simulink model "BANSHEE"  (Simulink 8.7)
settings: Solver=ode1  StartTime=0.0  StopTime=inf  FixedStep=Ts  MaxStep=1e-3  RelTol=1e-3
PostLoadFcn:
  | BANSHEE_init;
InitFcn:
  | BANSHEE_init;
values from neighbouring files (symbols this model uses):
  Ts = 100E-6    (= 0.0001)    [BANSHEE_init.m]
undefined symbols (not defined in the file or in its folder): Acid, Banshee_HWCtrl_IOs, Banshee_SEL751_Woodward_lib, DMS_slave_lib, DMSCommands, F1, F2, F3, fdesignblkfcn, Feeder1_lib, Feeder2_lib, Feeder3_lib, gcbh, generic_ethernet_cb, Lead, Left, relay_housing_lib, SM_UtilityService, SS_F1_RELAY_HOUSING, SS_F2_RELAY_HOUSING, SS_F3_RELAY_HOUSING, SS_Feeder1, SS_Feeder2, SS_Feeder3, SUBSTATION, TestSeq_slave_lib, TestSequenceCommands, type, utility_service_lib, V
libraries: powerlib x108, cables_lib x61, breaker_lib x53, rtio_generic_modbus x50, relay_modbus_lib x45, rtio_opalrt_op5142ex1 x37, transformer_lib x29, rteventslib x28, Load_lib x25, simulink x24, rtlab x20, ssn_lib x19
(part 6 of 9)

== system BANSHEE/SM_UtilityService/Banshee_HWCtrl_IOs/SEL-2440 FAST-LOAD-SHEDDING AND CB STATUS ==
  note: Breaker status
  note: CB202
      | CB203
      | CB301
      | CB302
      | CB303
      | CB304
      | spare
      | spare
  note: 751-1
      | 751-2
      | 751-3
      | CB101
      | CB102
      | CB103
      | CB108
      | CB201
  note: CB204
      | CB307
      | CB218
      | CB309
      | F1-GCB
      | CB205
      | CB211
      | F3-GCB
  note: CB104
      | CB107
      | CB206
      | CB208
      | CB212
      | CB308
      | CB114
      | CB219
  note: Copyright (c) 2016 Massachusetts Institute of Technology
      | Permission is hereby granted, free of charge, to any person obtaining a copy of this software and associated documentation files (the "Software"), to deal
      | in the Software without restriction, including without limitation the rights to use, copy, modify, merge, publish, distribute, sublicense, and/or sell copies of the
      | Software, and to permit persons to whom the Software is furnished to do so, subject to the following conditions:
      |
      | THE SOFTWARE IS PROVIDED "AS IS", WITHOUT WARRANTY OF ANY KIND, EXPRESS OR IMPLIED, INCLUDING BUT NOT LIMITED TO THE
      | WARRANTIES OF MERCHANTABILITY, FITNESS FOR A PARTICULAR PURPOSE AND NONINFRINGEMENT. IN NO EVENT SHALL THE AUTHORS
      | OR COPYRIGHT HOLDERS BE LIABLE FOR ANY CLAIM, DAMAGES OR OTHER LIABILITY, WHETHER IN AN ACTION OF CONTRACT, TORT OR
      | OTHERWISE, ARISING FROM, OUT OF OR IN CONNECTION WITH THE SOFTWARE OR THE USE OR OTHER DEALINGS IN THE SOFTWARE
  note: 16 bits to control (P, I load) breakers from Schwietzer
  CMBNE_SGNLS : Inport
  Bus Creator : BusCreator  Inputs=16
  Bus Selector : BusSelector  OutputSignals=F1_MS_IN.CB_DATA.F1_CB_4.Status,F1_MS_IN.CB_DATA.F1_CB_7.Status,F2_MS_IN.CB_DATA.F2_CB_6.Status,F2_MS_IN.CB_DATA.F2_CB_8.Status,F2_MS_IN.CB_DATA.F2_CB_12.Status,F3_MS_IN.CB_DATA.F3_CB_8.Status,F1_MS_IN.CB_DATA.F1_CB_14.Status,F2_MS_IN.CB_DATA.F2_CB_19.Status  OutputAsBus=on
  Bus Selector1 : BusSelector  OutputSignals=BESS_PV.EPC.BESS.BESS_MX1.cb_ms.Status,BESS_PV.EPC.PV.PV_MX1.cb_ms.Status
  Bus Selector6 : BusSelector  OutputSignals=F2_MS_IN.CB_DATA.F2_CB_4.Status,F3_MS_IN.CB_DATA.F3_CB_7.Status,F2_MS_IN.CB_DATA.F2_CB_18.Status,F3_MS_IN.CB_DATA.F3_CB_9.Status,F1_MS_IN.DIESEL_DATA.DIESEL_GCB.cb_ms.Status,F2_MS_IN.CB_DATA.F2_CB_5.Status,F2_MS_IN.CB_DATA.F2_CB_11.Status,F3_MS_IN.NG_CHP_DATA.NG_CHP_GCB.cb_ms.Status
  Bus Selector7 : BusSelector  OutputSignals=F1_MS_IN.CB_DATA.F1_PCC.Status,F2_MS_IN.CB_DATA.F2_PCC.Status,F3_MS_IN.CB_DATA.F3_PCC.Status,F1_MS_IN.CB_DATA.F1_CB_1.Status,F1_MS_IN.CB_DATA.F1_CB_2.Status,F1_MS_IN.CB_DATA.F1_CB_3.Status,F1_MS_IN.CB_DATA.F1_CB_8.Status,F2_MS_IN.CB_DATA.F2_CB_1.Status  OutputAsBus=on
  Bus Selector8 : BusSelector  OutputSignals=F2_MS_IN.CB_DATA.F2_CB_2.Status,F2_MS_IN.CB_DATA.F2_CB_3.Status,F3_MS_IN.CB_DATA.F3_CB_1.Status,F3_MS_IN.CB_DATA.F3_CB_2.Status,F3_MS_IN.CB_DATA.F3_CB_3.Status,F3_MS_IN.CB_DATA.F3_CB_4.Status
  Data Type Conversion : DataTypeConversion
  Data Type Conversion1 : DataTypeConversion
  Demux : Demux  Outputs=8
  Demux1 : Demux  Outputs=8
  Logical Operator : Logic  AllPortsSameDT=off  OutDataTypeStr=boolean
  Logical Operator1 : Logic  AllPortsSameDT=off  OutDataTypeStr=boolean
  Mux1 : Mux  Inputs=8
  Mux3 : Mux  Inputs=8
  OP5142EX1 DigitalIn : rtio_opalrt_op5142ex1/OP5142EX1 DigitalIn  CtrlName='OP5142EX1 Ctrl'  portNb=3  FcnNos=Slot 4 Module A Subsection 1  size=1  maxcount=8  count=8  sampleTime=0  numchan=8
      settings: AttributesFormatString=%<CtrlName>
  OP5142EX1 DigitalIn1 : rtio_opalrt_op5142ex1/OP5142EX1 DigitalIn  CtrlName='OP5142EX1 Ctrl'  portNb=4  FcnNos=Slot 4 Module A Subsection 2  size=1  maxcount=8  count=8  sampleTime=0  numchan=8
      settings: AttributesFormatString=%<CtrlName>
  OP5142EX1 DigitalOut : rtio_opalrt_op5142ex1/OP5142EX1 DigitalOut  CtrlName='OP5142EX1 Ctrl'  portNb=9  FcnNos=Slot 3 Module B Subsection 1  size=1  maxcount=8  count=8  numchan=8
      settings: AttributesFormatString=%<CtrlName>
  OP5142EX1 DigitalOut1 : rtio_opalrt_op5142ex1/OP5142EX1 DigitalOut  CtrlName='OP5142EX1 Ctrl'  portNb=10  FcnNos=Slot 3 Module B Subsection 2  size=1  maxcount=8  count=8  numchan=8
      settings: AttributesFormatString=%<CtrlName>
  OP5142EX1 DigitalOut2 : rtio_opalrt_op5142ex1/OP5142EX1 DigitalOut  CtrlName='OP5142EX1 Ctrl'  portNb=11  FcnNos=Slot 3 Module B Subsection 3  size=1  maxcount=8  count=8  numchan=8
      settings: AttributesFormatString=%<CtrlName>
  OP5142EX1 DigitalOut3 : rtio_opalrt_op5142ex1/OP5142EX1 DigitalOut  CtrlName='OP5142EX1 Ctrl'  portNb=12  FcnNos=Slot 3 Module B Subsection 4  size=1  maxcount=8  count=8  numchan=8
      settings: AttributesFormatString=%<CtrlName>
  Spares : Constant  Value=0
  Terminator1 : Terminator
  Terminator7 : Terminator
  SEL2440_FLS : Outport
  wires:
  [CMBNE_SGNLS] -> Bus Selector/1
  Bus Selector/1 -> OP5142EX1 DigitalOut/1
  Bus Selector8/1 -> Mux3/1  "<Status>"
  Bus Selector8/3 -> Mux3/3  "<Status>"
  Bus Selector8/2 -> Mux3/2  "<Status>"
  Bus Selector8/5 -> Mux3/5  "<Status>"
  Spares/1 -> Mux3/7, Mux3/8
  Bus Selector8/4 -> Mux3/4  "<Status>"
  Bus Selector7/1 -> OP5142EX1 DigitalOut2/1
  Bus Selector8/6 -> Mux3/6  "<Status>"
  Mux3/1 -> OP5142EX1 DigitalOut3/1
  OP5142EX1 DigitalIn/2 -> Terminator7/1
  OP5142EX1 DigitalIn1/2 -> Terminator1/1
  OP5142EX1 DigitalIn/1 -> Demux/1
  OP5142EX1 DigitalIn1/1 -> Demux1/1
  Demux/1 -> Bus Creator/1  "CB104"
  Demux/2 -> Bus Creator/2  "CB107"
  Demux/3 -> Bus Creator/3  "CB206"
  Demux/4 -> Bus Creator/4  "CB208"
  Demux/5 -> Bus Creator/5  "CB212"
  Demux/6 -> Bus Creator/6  "CB308"
  Demux/7 -> Bus Creator/7  "CB114"
  Demux/8 -> Bus Creator/8  "CB219"
  Demux1/7 -> Bus Creator/15
  Demux1/8 -> Bus Creator/16
  Demux1/6 -> Bus Creator/14
  Demux1/5 -> Bus Creator/13
  Demux1/4 -> Bus Creator/12  "CB309"
  Demux1/3 -> Bus Creator/11  "CB218"
  Demux1/2 -> Bus Creator/10  "CB307"
  Demux1/1 -> Bus Creator/9  "CB204"
  Bus Creator/1 -> SEL2440_FLS/1  "SEL2440_FLS"
  CMBNE_SGNLS/1 -> [CMBNE_SGNLS]
  [CMBNE_SGNLS] -> Bus Selector6/1
  [CMBNE_SGNLS] -> Bus Selector7/1
  [CMBNE_SGNLS] -> Bus Selector8/1
  [CMBNE_SGNLS] -> Bus Selector1/1
  Bus Selector1/1 -> [BESS_MX1_Status]  "<Status>"
  Bus Selector1/2 -> [PV_MX1_Status]  "<Status>"
  Bus Selector6/7 -> Logical Operator1/2  "<Status>"
  [PV_MX1_Status] -> Logical Operator1/1
  Bus Selector6/6 -> Logical Operator/2  "<Status>"
  [BESS_MX1_Status] -> Logical Operator/1
  Bus Selector6/5 -> Mux1/5  "<Status>"
  Bus Selector6/4 -> Mux1/4  "<Status>"
  Bus Selector6/3 -> Mux1/3  "<Status>"
  Bus Selector6/2 -> Mux1/2  "<Status>"
  Bus Selector6/1 -> Mux1/1  "<Status>"
  Logical Operator/1 -> Data Type Conversion/1
  Logical Operator1/1 -> Data Type Conversion1/1
  Bus Selector6/8 -> Mux1/8  "<Status>"
  Mux1/1 -> OP5142EX1 DigitalOut1/1
  Data Type Conversion/1 -> Mux1/6
  Data Type Conversion1/1 -> Mux1/7

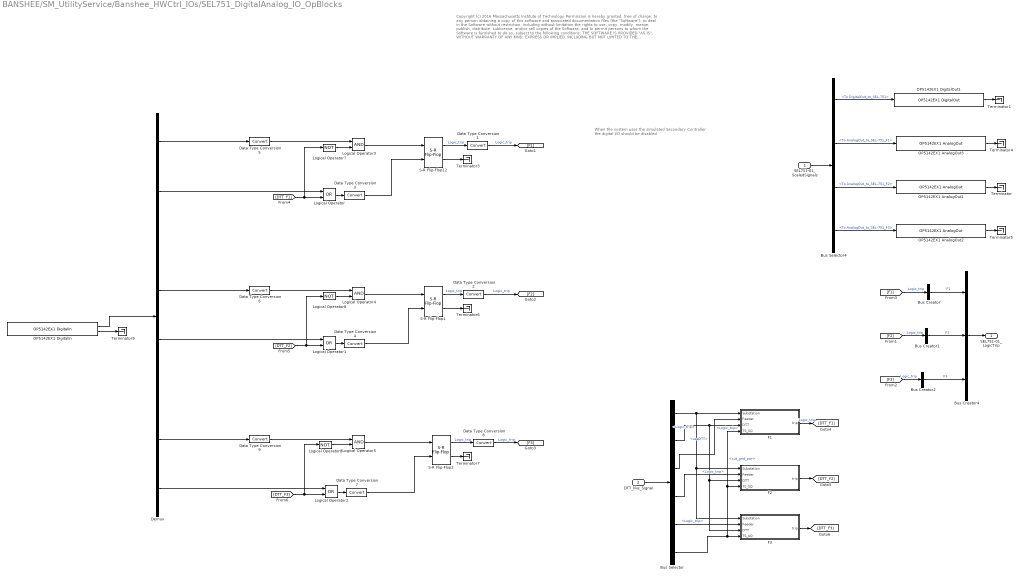
== system BANSHEE/SM_UtilityService/Banshee_HWCtrl_IOs/SEL751_DigitalAnalog_IO_OpBlocks ==
  note: When the system uses the simulated
      | Secondary Controller the digital I/O
      | should be disabled.
  note: Copyright (c) 2016 Massachusetts Institute of Technology
      | Permission is hereby granted, free of charge, to any person obtaining a copy of this software and associated documentation files (the "Software"), to deal
      | in the Software without restriction, including without limitation the rights to use, copy, modify, merge, publish, distribute, sublicense, and/or sell copies of the
      | Software, and to permit persons to whom the Software is furnished to do so, subject to the following conditions:
      |
      | THE SOFTWARE IS PROVIDED "AS IS", WITHOUT WARRANTY OF ANY KIND, EXPRESS OR IMPLIED, INCLUDING BUT NOT LIMITED TO THE
      | WARRANTIES OF MERCHANTABILITY, FITNESS FOR A PARTICULAR PURPOSE AND NONINFRINGEMENT. IN NO EVENT SHALL THE AUTHORS
      | OR COPYRIGHT HOLDERS BE LIABLE FOR ANY CLAIM, DAMAGES OR OTHER LIABILITY, WHETHER IN AN ACTION OF CONTRACT, TORT OR
      | OTHERWISE, ARISING FROM, OUT OF OR IN CONNECTION WITH THE SOFTWARE OR THE USE OR OTHER DEALINGS IN THE SOFTWARE
  SEL751-01_ScaledSignals : Inport
  DTT_like_Signal : Inport  Port=2
  Bus Creator : BusCreator  Inputs=1
  Bus Creator1 : BusCreator  Inputs=1
  Bus Creator2 : BusCreator  Inputs=1
  Bus Creator4 : BusCreator  Inputs=3
  Bus Selector : BusSelector  OutputSignals=SC_Signal.GridStatusCtrl.Substation.Logic_trip,SC_Signal.GridStatusCtrl.useDTT,SC_Signal.GridStatusCtrl.Grid_F1.Logic_trip,SC_Signal.GridStatusCtrl.Grid_F2.Logic_trip,SC_Signal.GridStatusCtrl.Grid_F3.Logic_trip,cut_grid_pwr
  Bus Selector4 : BusSelector  OutputSignals=To DigitalOut_to_SEL-751,To AnalogOut_to_SEL-751_F1,To AnalogOut_to_SEL-751_F2,To AnalogOut_to_SEL-751_F3
  Data Type Conversion{1..9} (9 alike) : DataTypeConversion
  Demux : Demux  Outputs=8
  F1 : Subsystem
  F2 : Subsystem
  F3 : Subsystem
  Logical Operator : Logic  Operator=OR  AllPortsSameDT=off  OutDataTypeStr=boolean
  Logical Operator1 : Logic  Operator=OR  AllPortsSameDT=off  OutDataTypeStr=boolean
  Logical Operator2 : Logic  Operator=OR  AllPortsSameDT=off  OutDataTypeStr=boolean
  Logical Operator3 : Logic  AllPortsSameDT=off  OutDataTypeStr=boolean
  Logical Operator4 : Logic  AllPortsSameDT=off  OutDataTypeStr=boolean
  Logical Operator5 : Logic  AllPortsSameDT=off  OutDataTypeStr=boolean
  Logical Operator6 : Logic  Operator=NOT  AllPortsSameDT=off  OutDataTypeStr=boolean
  Logical Operator7 : Logic  Operator=NOT  AllPortsSameDT=off  OutDataTypeStr=boolean
  Logical Operator8 : Logic  Operator=NOT  AllPortsSameDT=off  OutDataTypeStr=boolean
  OP5142EX1 AnalogOut1 : rtio_opalrt_op5142ex1/OP5142EX1 AnalogOut  CtrlName='OP5142EX1 Ctrl'  portNb=2  FcnNos=Slot 1 Module A Subsection 2  size=16  maxcount=8  count=8  numchan=8  israngeinput=off  voltagerange=[-16 ... 16]  slot=0  side=0  mismatch=0  slotside=Slot_1_Module_A
      settings: AttributesFormatString=%<CtrlName>
  OP5142EX1 AnalogOut2 : rtio_opalrt_op5142ex1/OP5142EX1 AnalogOut  CtrlName='OP5142EX1 Ctrl'  portNb=3  FcnNos=Slot 2 Module A Subsection 1  size=16  maxcount=8  count=8  numchan=8  israngeinput=off  voltagerange=[-16 ... 16]  slot=1  side=0  mismatch=0  slotside=Slot_2_Module_A
      settings: AttributesFormatString=%<CtrlName>
  OP5142EX1 AnalogOut3 : rtio_opalrt_op5142ex1/OP5142EX1 AnalogOut  CtrlName='OP5142EX1 Ctrl'  portNb=1  FcnNos=Slot 1 Module A Subsection 1  size=16  maxcount=8  count=8  numchan=8  israngeinput=off  voltagerange=[-16 ... 16]  slot=0  side=0  mismatch=0  slotside=Slot_1_Module_A
      settings: AttributesFormatString=%<CtrlName>
  OP5142EX1 DigitalIn : rtio_opalrt_op5142ex1/OP5142EX1 DigitalIn  CtrlName='OP5142EX1 Ctrl'  portNb=5  FcnNos=Slot 4 Module A Subsection 3  size=1  maxcount=8  count=8  sampleTime=0  numchan=8
      settings: AttributesFormatString=%<CtrlName>
  OP5142EX1 DigitalOut1 : rtio_opalrt_op5142ex1/OP5142EX1 DigitalOut  CtrlName='OP5142EX1 Ctrl'  portNb=13  FcnNos=Slot 4 Module B Subsection 1  size=1  maxcount=8  count=8  numchan=8
      settings: AttributesFormatString=%<CtrlName>
  S-R Flip-Flop1 : simulink_extras/Flip Flops/S-R Flip-Flop  initial_condition=1
  S-R Flip-Flop12 : simulink_extras/Flip Flops/S-R Flip-Flop  initial_condition=1
  S-R Flip-Flop2 : simulink_extras/Flip Flops/S-R Flip-Flop  initial_condition=1
  Terminator{,1,3..7,9} (8 alike) : Terminator
  SEL751-01_LogicTrip : Outport
  wires:
  Data Type Conversion1/1 -> [F1]  "Logic_trip"
  Bus Creator4/1 -> SEL751-01_LogicTrip/1
  Data Type Conversion2/1 -> [F2]  "Logic_trip"
  Data Type Conversion8/1 -> [F3]  "Logic_trip"
  Bus Creator/1 -> Bus Creator4/1  "F1"
  Bus Creator2/1 -> Bus Creator4/3  "F3"
  Bus Creator1/1 -> Bus Creator4/2  "F2"
  OP5142EX1 DigitalOut1/1 -> Terminator1/1
  OP5142EX1 AnalogOut1/1 -> Terminator/1
  Bus Selector4/1 -> OP5142EX1 DigitalOut1/1  "<To DigitalOut_to_SEL-751>"
  SEL751-01_ScaledSignals/1 -> Bus Selector4/1
  OP5142EX1 AnalogOut2/1 -> Terminator5/1
  OP5142EX1 AnalogOut3/1 -> Terminator4/1
  S-R Flip-Flop1/1 -> Data Type Conversion2/1  "Logic_trip"
  S-R Flip-Flop12/1 -> Data Type Conversion1/1  "Logic_trip"
  S-R Flip-Flop2/1 -> Data Type Conversion8/1  "Logic_trip"
  Bus Selector4/4 -> OP5142EX1 AnalogOut2/1  "<To AnalogOut_to_SEL-751_F3>"
  Bus Selector4/3 -> OP5142EX1 AnalogOut1/1  "<To AnalogOut_to_SEL-751_F2>"
  Bus Selector4/2 -> OP5142EX1 AnalogOut3/1  "<To AnalogOut_to_SEL-751_F1>"
  Demux/1 -> Data Type Conversion5/1
  Data Type Conversion3/1 -> S-R Flip-Flop12/2
  Demux/7 -> Data Type Conversion9/1
  OP5142EX1 DigitalIn/2 -> Terminator9/1
  S-R Flip-Flop12/2 -> Terminator3/1
  S-R Flip-Flop1/2 -> Terminator6/1
  S-R Flip-Flop2/2 -> Terminator7/1
  DTT_like_Signal/1 -> Bus Selector/1
  [F1] -> Bus Creator/1  "Logic_trip"
  [F2] -> Bus Creator1/1  "Logic_trip"
  [F3] -> Bus Creator2/1  "Logic_trip"
  Bus Selector/1 -> F2/1(Substation), F3/1(Substation), F1/1(Substation)  "<Logic_trip>"
  Bus Selector/2 -> F3/3(DTT), F2/3(DTT), F1/3(DTT)  "<useDTT>"
  Bus Selector/3 -> F1/2(Feeder)  "<Logic_trip>"
  Bus Selector/4 -> F2/2(Feeder)  "<Logic_trip>"
  Bus Selector/5 -> F3/2(Feeder)  "<Logic_trip>"
  F1/1(trip) -> [DTT_F1]  "Logic_trip"
  F2/1(trip) -> [DTT_F2]
  F3/1(trip) -> [DTT_F3]
  [DTT_F1] -> Logical Operator7/1, Logical Operator/2
  Logical Operator/1 -> Data Type Conversion3/1
  [DTT_F2] -> Logical Operator6/1, Logical Operator1/2
  Logical Operator1/1 -> Data Type Conversion4/1
  [DTT_F3] -> Logical Operator8/1, Logical Operator2/2
  Logical Operator2/1 -> Data Type Conversion7/1
  Data Type Conversion4/1 -> S-R Flip-Flop1/2
  Data Type Conversion7/1 -> S-R Flip-Flop2/2
  Bus Selector/6 -> F1/4(TS_SQ), F2/4(TS_SQ), F3/4(TS_SQ)  "<cut_grid_pwr>"
  Demux/2 -> Logical Operator/1
  Demux/4 -> Data Type Conversion6/1
  Demux/5 -> Logical Operator1/1
  Demux/8 -> Logical Operator2/1
  OP5142EX1 DigitalIn/1 -> Demux/1
  Data Type Conversion9/1 -> Logical Operator5/1
  Data Type Conversion6/1 -> Logical Operator4/1
  Data Type Conversion5/1 -> Logical Operator3/1
  Logical Operator7/1 -> Logical Operator3/2
  Logical Operator8/1 -> Logical Operator5/2
  Logical Operator6/1 -> Logical Operator4/2
  Logical Operator5/1 -> S-R Flip-Flop2/1
  Logical Operator4/1 -> S-R Flip-Flop1/1
  Logical Operator3/1 -> S-R Flip-Flop12/1

== system BANSHEE/SM_UtilityService/Banshee_HWCtrl_IOs/Woodward Inputs ==
  note: Copyright (c) 2016 Massachusetts Institute of Technology
      | Permission is hereby granted, free of charge, to any person obtaining a copy of this software and associated documentation files (the "Software"), to deal
      | in the Software without restriction, including without limitation the rights to use, copy, modify, merge, publish, distribute, sublicense, and/or sell copies of the
      | Software, and to permit persons to whom the Software is furnished to do so, subject to the following conditions:
      |
      | THE SOFTWARE IS PROVIDED "AS IS", WITHOUT WARRANTY OF ANY KIND, EXPRESS OR IMPLIED, INCLUDING BUT NOT LIMITED TO THE
      | WARRANTIES OF MERCHANTABILITY, FITNESS FOR A PARTICULAR PURPOSE AND NONINFRINGEMENT. IN NO EVENT SHALL THE AUTHORS
      | OR COPYRIGHT HOLDERS BE LIABLE FOR ANY CLAIM, DAMAGES OR OTHER LIABILITY, WHETHER IN AN ACTION OF CONTRACT, TORT OR
      | OTHERWISE, ARISING FROM, OUT OF OR IN CONNECTION WITH THE SOFTWARE OR THE USE OR OTHER DEALINGS IN THE SOFTWARE
  note: GR1 A AOUT (CH00-15)
  note: All signals should be scaled accordingly prior connecting to this block
  Generator1_Voltage : Inport
  Generator1_Current : Inport  Port=2
  Mains1_Voltage : Inport  Port=3
  Mains1_Current : Inport  Port=4
  MPU1_speed : Inport  Port=5
  Generator2_Voltage : Inport  Port=6
  Generator2_Current : Inport  Port=7
  Mains2_Voltage : Inport  Port=8
  Mains2_Current : Inport  Port=9
  MPU2_speed : Inport  Port=10
  AnalogOut : rtio_opalrt_common/AnalogOut  CtrlName='OpCtrl'  portNb=1  FcnNos=Slot 1 Module A Subsection 1  size=16  maxcount=8  count=8  numchan=8  israngeinput=off  voltagerange=[-16 ... 16]  slot=0  side=0  mismatch=0  slotside=Slot_1_Module_A
      settings: AttributesFormatString=%<CtrlName>
  AnalogOut1 : rtio_opalrt_common/AnalogOut  CtrlName='OpCtrl'  portNb=2  FcnNos=Slot 1 Module A Subsection 2  size=16  maxcount=8  count=8  numchan=8  israngeinput=off  voltagerange=[-16 ... 16]  slot=0  side=0  mismatch=0  slotside=Slot_1_Module_A
      settings: AttributesFormatString=%<CtrlName>
  AnalogOut2 : rtio_opalrt_common/AnalogOut  CtrlName='OpCtrl'  portNb=3  FcnNos=Slot 2 Module A Subsection 1  size=16  maxcount=8  count=8  numchan=8  israngeinput=off  voltagerange=[-16 ... 16]  slot=1  side=0  mismatch=0  slotside=Slot_2_Module_A
      settings: AttributesFormatString=%<CtrlName>
  AnalogOut3 : rtio_opalrt_common/AnalogOut  CtrlName='OpCtrl'  portNb=4  FcnNos=Slot 2 Module A Subsection 2  size=16  maxcount=8  count=8  numchan=8  israngeinput=off  voltagerange=[-16 ... 16]  slot=1  side=0  mismatch=0  slotside=Slot_2_Module_A
      settings: AttributesFormatString=%<CtrlName>
  Demux : Demux  Outputs=2
  Demux{1..5,7..9} (8 alike) : Demux  Outputs=3
  Demux6 : Demux  Outputs=2
  Mux{,1,3..4} (4 alike) : Mux  Inputs=8
  Mux2 : Mux  Inputs=2
  Mux5 : Mux  Inputs=2
  Terminator{,1..3} (4 alike) : Terminator
  wires:
  Mains1_Voltage/1 -> Demux2/1
  Generator1_Voltage/1 -> Demux1/1
  Mux2/1 -> Demux/1
  Mux1/1 -> Mux2/2
  Mux/1 -> Mux2/1
  Demux/2 -> AnalogOut1/1
  Demux/1 -> AnalogOut/1
  AnalogOut1/1 -> Terminator1/1
  AnalogOut/1 -> Terminator/1
  Demux1/1 -> Mux/1
  Demux1/2 -> Mux/2
  Demux1/3 -> Mux/3
  Demux2/1 -> Mux/4
  Demux2/2 -> Mux/5
  Demux2/3 -> Mux/6
  MPU1_speed/1 -> Mux1/5
  Demux4/1 -> Mux/7
  Demux4/2 -> Mux/8
  Demux4/3 -> Mux1/1
  Demux5/1 -> Mux1/2
  Demux5/2 -> Mux1/3
  Demux5/3 -> Mux1/4
  Mux5/1 -> Demux6/1
  Mux4/1 -> Mux5/2
  Mux3/1 -> Mux5/1
  Demux6/2 -> AnalogOut3/1
  Demux6/1 -> AnalogOut2/1
  AnalogOut3/1 -> Terminator3/1
  AnalogOut2/1 -> Terminator2/1
  Generator1_Current/1 -> Demux3/1
  Demux3/1 -> Mux3/2
  Demux3/2 -> Mux3/3
  Demux3/3 -> Mux3/4
  Mains1_Current/1 -> Demux7/1
  Demux7/1 -> Mux3/1
  Mains2_Voltage/1 -> Demux5/1
  Generator2_Voltage/1 -> Demux4/1
  MPU2_speed/1 -> Mux1/6
  Mains2_Current/1 -> Demux8/1
  Demux8/1 -> Mux3/5
  Generator2_Current/1 -> Demux9/1
  Demux9/1 -> Mux3/6
  Demux9/2 -> Mux3/7
  Demux9/3 -> Mux3/8

== system BANSHEE/SM_UtilityService/Banshee_HWCtrl_IOs/Woodward Outputs - Diesel - Gen2 ==
  note: Copyright (c) 2016 Massachusetts Institute of Technology
      | Permission is hereby granted, free of charge, to any person obtaining a copy of this software and associated documentation files (the "Software"), to deal
      | in the Software without restriction, including without limitation the rights to use, copy, modify, merge, publish, distribute, sublicense, and/or sell copies of the
      | Software, and to permit persons to whom the Software is furnished to do so, subject to the following conditions:
      |
      | THE SOFTWARE IS PROVIDED "AS IS", WITHOUT WARRANTY OF ANY KIND, EXPRESS OR IMPLIED, INCLUDING BUT NOT LIMITED TO THE
      | WARRANTIES OF MERCHANTABILITY, FITNESS FOR A PARTICULAR PURPOSE AND NONINFRINGEMENT. IN NO EVENT SHALL THE AUTHORS
      | OR COPYRIGHT HOLDERS BE LIABLE FOR ANY CLAIM, DAMAGES OR OTHER LIABILITY, WHETHER IN AN ACTION OF CONTRACT, TORT OR
      | OTHERWISE, ARISING FROM, OUT OF OR IN CONNECTION WITH THE SOFTWARE OR THE USE OR OTHER DEALINGS IN THE SOFTWARE
  Gen2 MCB Status : Inport
  WoodwardBias : Inport  Port=2
  Bus Creator1 : BusCreator  Inputs=1
  DIO - Gr3 : Subsystem
  DIO - Woodward : Subsystem
  DOUT type config : Subsystem
  Woodward Primary Inputs - Gen2 : Subsystem
  Digital Inputs : Outport
  Gen2 Gov and AVR : Outport  Port=2
  Gen2 Fuel Enable : Outport  Port=3
  Gen2 GCB : Outport  Port=4
  Gen2 MCB : Outport  Port=5
  wires:
  Bus Creator1/1 -> Digital Inputs/1
  DIO - Woodward/1(DIn1) -> DIO - Gr3/1(Dout)
  DIO - Gr3/1(DIn) -> Bus Creator1/1, DIO - Woodward/1(Din_Wood)  "DIN"
  Woodward Primary Inputs - Gen2/1(Gen2 Gov and AVR) -> Gen2 Gov and AVR/1
  DIO - Woodward/3(Gen2 GCB) -> Gen2 GCB/1
  DIO - Woodward/2(Gen2 Fuel Enable) -> Gen2 Fuel Enable/1
  DIO - Woodward/4(Gen2 MCB) -> Gen2 MCB/1
  Gen2 MCB Status/1 -> DIO - Woodward/2(Gen2 MCB Status)
  WoodwardBias/1 -> Woodward Primary Inputs - Gen2/1(WoodwardBias)

== system BANSHEE/SM_UtilityService/Banshee_HWCtrl_IOs/Woodward Outputs - NGCHP - Gen1 ==
  note: Copyright (c) 2016 Massachusetts Institute of Technology
      | Permission is hereby granted, free of charge, to any person obtaining a copy of this software and associated documentation files (the "Software"), to deal
      | in the Software without restriction, including without limitation the rights to use, copy, modify, merge, publish, distribute, sublicense, and/or sell copies of the
      | Software, and to permit persons to whom the Software is furnished to do so, subject to the following conditions:
      |
      | THE SOFTWARE IS PROVIDED "AS IS", WITHOUT WARRANTY OF ANY KIND, EXPRESS OR IMPLIED, INCLUDING BUT NOT LIMITED TO THE
      | WARRANTIES OF MERCHANTABILITY, FITNESS FOR A PARTICULAR PURPOSE AND NONINFRINGEMENT. IN NO EVENT SHALL THE AUTHORS
      | OR COPYRIGHT HOLDERS BE LIABLE FOR ANY CLAIM, DAMAGES OR OTHER LIABILITY, WHETHER IN AN ACTION OF CONTRACT, TORT OR
      | OTHERWISE, ARISING FROM, OUT OF OR IN CONNECTION WITH THE SOFTWARE OR THE USE OR OTHER DEALINGS IN THE SOFTWARE
  Gen1 MCB Status : Inport
  WoodwardBias : Inport  Port=2
  Bus Creator1 : BusCreator  Inputs=1
  DIO - Gr3 : Subsystem
  DIO - Woodward : Subsystem
  DOUT type config : Subsystem
  Woodward Primary Inputs - Gen1 : Subsystem
  Digital Inputs : Outport
  Gen1 Gov and AVR : Outport  Port=2
  Gen1 Fuel Enable : Outport  Port=3
  Gen1 GCB : Outport  Port=4
  Gen1 MCB : Outport  Port=5
  wires:
  DIO - Woodward/4(DIn1) -> DIO - Gr3/1(Dout)
  DIO - Gr3/1(DIn) -> DIO - Woodward/1(Din_Wood), Bus Creator1/1  "DIN"
  Bus Creator1/1 -> Digital Inputs/1
  Woodward Primary Inputs - Gen1/1(Gen1 Gov and AVR) -> Gen1 Gov and AVR/1
  WoodwardBias/1 -> Woodward Primary Inputs - Gen1/1(WoodwardBias)
  DIO - Woodward/2(Gen1 GCB) -> Gen1 GCB/1
  DIO - Woodward/3(Gen1 MCB) -> Gen1 MCB/1
  DIO - Woodward/1(Gen1 Fuel Enable) -> Gen1 Fuel Enable/1
  Gen1 MCB Status/1 -> DIO - Woodward/2(Gen1 MCB Status)

== system BANSHEE/SM_UtilityService/Number of seconds of recording/Increment ==
  Trigger : TriggerPort  VariantControl=Variant
  Increment : Constant
  Memory : Memory  InheritSampleTime=on
  Sum : Sum  Inputs=|++
  Out1 : Outport
  wires:
  Increment/1 -> Sum/2
  Memory/1 -> Sum/1
  Sum/1 -> Memory/1, Out1/1

== system BANSHEE/SS_F3_RELAY_HOUSING/Banshee UDP Data - Formatted Packets/Ethernet communication interface ==
  note: Ethernet communication interface example model
  Data trigger : Inport
  Data to send : Inport  Port=2
  AsyncEthernetCtrl : S-Function  InitFcn=generic_ethernet_cb('initfcn');  FunctionName=sfun_gen_async_ctrl  Parameters=ctrl_id, nbr_to_remote_endpoint, type_to_remote_endpoint,nbr_from_remote_endpoint,type_from_remote_endpoint,protocol,tcp_mode, port, offset_to_remote_endpoint,offset_from_remote_endpoint,swap_tx,swap_rx,0,nic_name,remote_ip,'','','','','','','','','','',exe_name,0  SFunctionDeploymentMode=off  EnableBusSupport=off  mask(AsyncEthernetCtrl){ctrl_id=1, nbr_to_remote_endpoint=375, type_to_remote_endpoint=INT32, offset_to_remote_endpoint=0, nbr_from_remote_endpoint=4, type_from_remote_endpoint=DOUBLE, offset_from_remote_endpoint=0, nic_name=eth0, protocol=UDP, tcp_mode=Server, port=7200, remote_ip=255.255.255.255, exe_name=AsyncEthernet, swap_tx=off, swap_rx=off}
      mask prompts: ctrl_id "Controller ID"; nbr_to_remote_endpoint "Number of data to send"; type_to_remote_endpoint "Type of data to send"; offset_to_remote_endpoint "Byte offset of transmission buffer"; nbr_from_remote_endpoint "Number of data expected to be received"; type_from_remote_endpoint "Type of data expected to be received"; offset_from_remote_endpoint "Byte offset of reception buffer"; nic_name "Network interface name"; tcp_mode "TCP mode"; remote_ip "Remote IP address"; exe_name "Name of the executable"; swap_tx "Swap data endianness before transmission"; swap_rx "Swap data endianness after reception"
      mask help: Generic asynchronous process configuration block
      mask Help: eval('rtlab_help(''opasyncgenctrl'');');
      mask TypeOptions type_to_remote_endpoint: UINT8 | INT8 | UINT16 | INT16 | UINT32 | INT32 | FLOAT | DOUBLE
      mask TypeOptions type_from_remote_endpoint: UINT8 | INT8 | UINT16 | INT16 | UINT32 | INT32 | FLOAT | DOUBLE
      mask TypeOptions protocol: UDP | TCP
      mask TypeOptions tcp_mode: Client | Server
      mask Display: disp(sprintf('\nEthernet communication \ninterface controller\n'))
  B-width : SignalSpecification  Dimensions=nbr_from_remote_endpoint
  Constant : Constant  Value=1000
  Logo : opal_lib/Logo1  vide=[]
  Mux : Mux  Inputs=2
  OpAsyncRecv : rtlab/Communication/Asynchronous/OpAsyncRecv  ctl_id=ctrl_id  recv_id=ctrl_id  enable_param=off  fp1=1  fp2=2  fp3=3  fp4=4  fp5=5  sp1=string1  sp2=string2  sp3=string3  sp4=string4  sp5=string5
  OpAsyncSend : rtlab/Communication/Asynchronous/OpAsyncSend  ctl_id=ctrl_id  send_id=ctrl_id  mode=DONT_NEED_REPLY  enable_param=off  fp1=1  fp2=2  fp3=3  fp4=4  fp5=5  sp1=string1  sp2=string2  sp3=string3  sp4=string4  sp5=string5
  Terminator : Terminator
  Data received : Outport
  Status : Outport  Port=2
  wires:
  Data to send/1 -> OpAsyncSend/2
  Data trigger/1 -> OpAsyncSend/1
  OpAsyncSend/1 -> Mux/1
  OpAsyncRecv/1 -> Mux/2
  Mux/1 -> Status/1
  Constant/1 -> OpAsyncRecv/1
  OpAsyncRecv/2 -> Terminator/1
  OpAsyncRecv/3 -> B-width/1
  B-width/1 -> Data received/1

== system BANSHEE/SS_PV_BESS/EPC/Contactors1 ==
  note: with 10ohm resistor
  note: changed to 1000
      | to slow down the time
  Precharge : Inport
  Main Contactor : Inport  Port=2
  Brk_Battery : powerlib/Power Electronics/Ideal Switch  Ron=0.001  Lon=0  IC=0  Rs=1e6  Cs=inf  Measurements=on
  Brk_Precharge : powerlib/Power Electronics/Ideal Switch  Ron=1  Lon=0  IC=0  Rs=1e6  Cs=inf  Measurements=on
  DC+ Source : PMIOPort  Port=1  Side=Right
  DC+ Bus : PMIOPort  Port=2  Side=Left
  DC- Source : PMIOPort  Port=3  Side=Left
  DC- Bus : PMIOPort  Port=4  Side=Right
  wires:
  Precharge/1 -> Brk_Precharge/1
  Main Contactor/1 -> Brk_Battery/1
  connections:
  Brk_Battery/LConn1 -- DC+ Bus/RConn1 -- Brk_Precharge/LConn1
  Brk_Battery/RConn1 -- DC+ Source/RConn1 -- Brk_Precharge/RConn1
  DC- Bus/RConn1 -- DC- Source/RConn1

== system BANSHEE/SS_PV_BESS/EPC/Contactors2 ==
  note: with 10ohm resistor
  note: changed to 1000
      | to slow down the time
  Precharge : Inport
  Main Contactor : Inport  Port=2
  Brk_Battery : powerlib/Power Electronics/Ideal Switch  Ron=0.001  Lon=0  IC=0  Rs=1e6  Cs=inf  Measurements=on
  Brk_Precharge : powerlib/Power Electronics/Ideal Switch  Ron=1  Lon=0  IC=0  Rs=1e6  Cs=inf  Measurements=on
  DC+ Source : PMIOPort  Port=1  Side=Right
  DC+ Bus : PMIOPort  Port=2  Side=Left
  DC- Source : PMIOPort  Port=3  Side=Left
  DC- Bus : PMIOPort  Port=4  Side=Right
  wires:
  Precharge/1 -> Brk_Precharge/1
  Main Contactor/1 -> Brk_Battery/1
  connections:
  Brk_Battery/LConn1 -- DC+ Bus/RConn1 -- Brk_Precharge/LConn1
  Brk_Battery/RConn1 -- DC+ Source/RConn1 -- Brk_Precharge/RConn1
  DC- Bus/RConn1 -- DC- Source/RConn1

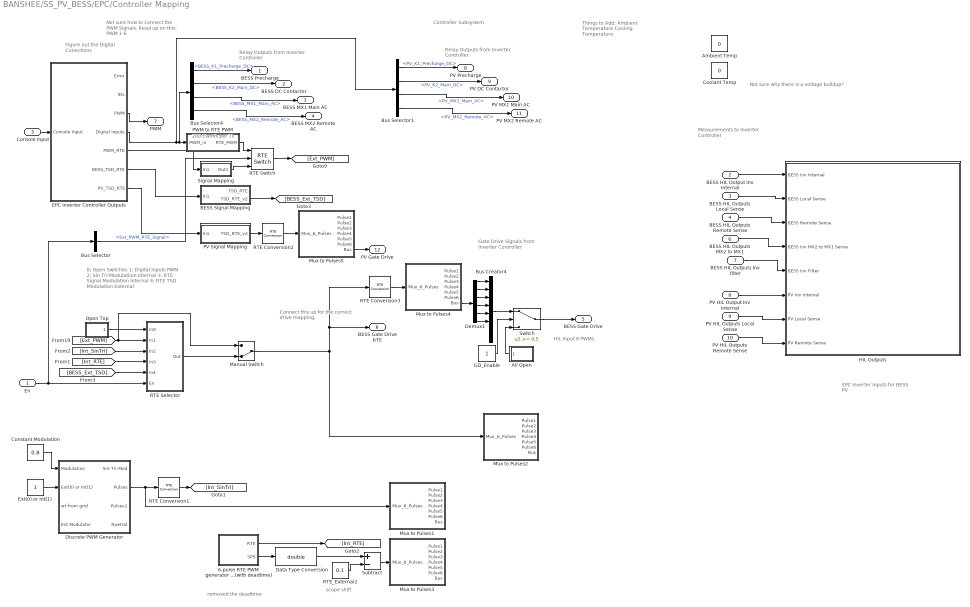
== system BANSHEE/SS_PV_BESS/EPC/Controller Mapping ==
  note: Relay Outputs from
      | Inverter Controller
  note: Controller Subsystem
  note: Gate Drive Signals from
      | Inverter Controller
  note: Relay Outputs from
      | Inverter Controller
  note: Measurements to
      | Inverter Controller
  note: Not sure why there is a voltage buildup?
  note: Things to Add:
      | Ambient Temperature
      | Cooling Temperature
  note: HIL Input
      | 8 PWMs
  note: Not sure how to connect
      | the PWM Signals.
      | Read up on this.
      | PWM 1-6
  note: Figure out the
      | Digital Conections
  note: removed the deadtime
  note: scope shift
  note: 0; Open Switches
      | 1: Digital Inputs PWM
      | 2: Sin Tri Modulatiion Internal
      | 3: RTE Signal Modulation Internal
      | 4: RTE TSD Modulation External
  note: 200 Events per Ts
  note: Connect this
      | up for the
      | correct drive
      | mapping.
  note: EPC Inverter Inputs for
      | BESS
      | PV
  En : Inport
  "BESS HIL Output Inv Internal " : Inport  Port=2
  BESS HIL Outputs Local Sense : Inport  Port=3
  BESS HIL Outputs Remote Sense : Inport  Port=4
  Console Input : Inport  Port=5
  BESS HIL Outputs MX2 to MX1 : Inport  Port=6
  BESS HIL Outputs Inv filter : Inport  Port=7
  "PV HIL Output Inv Internal " : Inport  Port=8
  PV HIL Outputs Local Sense : Inport  Port=9
  PV HIL Outputs Remote Sense : Inport  Port=10
  6-pulse RTE PWM generator (with deadtime) : Subsystem  Tag=RTEcontrol_s38shd7k88  AncestorBlock=|  mask(3-phase RT-Event Discrete PWM Generator){GeneratorMode=3-arm  bridge (6 pulses), Fc=5000, Ts=Ts, mIndex=0.9, Freq=60, Phase=0, Tdead=0}
      | artemis/Tools /Rt-Event 
      | control blocks/6-pulse RTE
      | PWM generator
      | (with deadtime)
      mask prompts: GeneratorMode "Generator Mode"; Fc "Carrier frequency (Hz):"; Ts "Sample time:"; mIndex "Modulation index  (0<m<1) :"; Freq "Frequency of output voltage (Hz)"; Phase "Phase of output voltage (degrees)"; Tdead "Deadtime (s)"
      mask help:
      | This  block generates RT-Event pulses for 3-phase discrete time compensated  carrier-based PWM (Pulse Width Modulation), self-commutated IGBTs,GTOs or FETs bridges in ARTEMIS-RTE.
      |
      | RT-Event pulses are pair of signals that contain the logical value of the switch {on.off} and a timing value used in ARTEMIS-RTE to compensate for in-step switching actions.
      | PSB pulses consist of the logicla part only.
      |
      | Pulses 1,3 and 5 are respectively for the upper switches of the first,second and third arm. Pulses 2,4 and 6 are for the lower switches.
      mask init:
      | set_param(gcb,'LinkStatus','inactive');
      | if Freq==0
      |     Phase=90;
      | end
      |     Internal_Phase=[0 -2*pi/3 2*pi/3];
      |     Signal_PortWidth=3;
      |     Select1_Elements=[1 4 2 5 3 6];
      |     Select1_PortWidth=6;
      |    Select3_Elements=[1 2 3 4 5 6];
      |    Select3_PortWidth=12;
      mask TypeOptions GeneratorMode: 3-arm  bridge (6 pulses)
      mask Display: plot(0,0,100,100,[60,57,57,56,56,53,53,50,50,47,47,41,41,38,38,35,35,32,32,31,31,25,25,24,24,22,22,19,19,16,16,11,11,8,8,5,5,3,3,2,2,0],[20,20,80,80,20,20,80,80,20,20,80,80,20,20,80,80,20,20,80,80,20,20,80,80,20,20,80,80,20,20,80,80,20,20,80,80,20,20,80,80,20,20])
  All Open : Subsystem
  Ambient Temp : Constant  Value=0
  BESS Signal Mapping : Subsystem
  Bus Creator4 : BusCreator  Inputs=8
  Bus Selector : BusSelector  OutputSignals=Ext_PWM_RTE_Signal
  Bus Selector1 : BusSelector  OutputSignals=DIN.DI_CH00-07.PV_K1_Precharge_DC,DIN.DI_CH00-07.PV_K2_Main_DC,DIN.DI_CH00-07.PV_MX1_Main_AC,DIN.DI_CH00-07.PV_MX2_Remote_AC
  Bus Selector4 : BusSelector  OutputSignals=DIN.DI_CH00-07.BESS_K1_Precharge_DC,DIN.DI_CH00-07.BESS_K2_Main_DC,DIN.DI_CH00-07.BESS_MX1_Main_AC,DIN.DI_CH00-07.BESS_MX2_Remote_AC
  Constant Modulation : Constant  Value=0.8
  Coolant Temp : Constant  Value=0
  Data Type Conversion : DataTypeConversion  OutDataTypeStr=double
  Demux1 : Demux  Outputs=6
  Discrete PWM Generator : Subsystem  AncestorBlock=|  DialogController=POWERSYS.PowerSysDialog  mask(Discrete PWM Generator){GeneratorMode=3-arm  bridge (6 pulses), Fc=5000, Ts=Ts, Internal=on, mIndex=0.8, Freq=60, Phase=0}
      | powerlib_extras/Discrete 
      | Control Blocks/Discrete
      | PWM Generator
      mask prompts: GeneratorMode "Generator Mode"; Fc "Carrier frequency (Hz):"; Ts "Sample time:"; Internal "Internal generation of modulating signal(s)"; mIndex "Modulation index  (0<m<1) :"; Freq "Frequency of output voltage (Hz)"; Phase "Phase of output voltage (degrees)"
      mask help:
      | This discrete block generates pulses for carrier-based PWM (Pulse Width Modulation), self-commutated IGBTs,GTOs or FETs bridges.
      |
      | Depending on the number of bridge arms selected in the "Generator Mode" parameter, the block can be used either for single-phase or three-phase PWM control.
      mask init:
      | powericon('psbcallbacks',gcb,'Discrete PWM Generator');
      | if Freq==0
      |     Phase=90;
      | end
      | switch GeneratorMode
      | case 1,
      |     Internal_Phase=0;
      |    Signal_PortWidth=1;
      |    Select1_Elements=[1 2];
      |    Select1_PortWidth=2;
      |    Select3_Elements=[1 2];
      |    Select3_PortWidth=4;
      | case 2,
      |     Internal_Phase=0;
      |     Signal_PortWidth=1;
      |     Select1_Elements=[1 2];
      |     Select1_PortWidth=2;
      |     Select3_Elements=[1 2 3 4];
      |     Select3_PortWidth=4;
      | case 3,
      |     Internal_Phase=[0 -2*pi/3 2*pi/3];
      |     Signal_PortWidth=3;
      |     Select1_Elements=[1 4 2 5 3 6];
      |     Select1_PortWidth=6;
      |    Select3_Elements=[1 2 3 4 5 6];
      |    Select3_PortWidth=12;
      | case 4,
      |     Internal_Phase=[0 -2*pi/3 2*pi/3];
      |     Signal_PortWidth=3;
      |     Select1_Elements=[1 4 2 5 3 6];
      |     Select1_PortWidth=6;
      |    Select3_Elements=[1 2 3 4 5 6 7 8 9 10 11 12];
      |    Select3_PortWidth=12;
      | end
      | power_initmask();
      mask Help:
      | The output pulses are a vector (with values=0 or 1). Depending on the selected "Generator Mode", the output vector contains:
      | For a 1-arm  bridge: Two pulses. Pulse 1 is for the upper switch and pulse 2 is for the lower switch.
      | For a 2-arm  bridge: Four pulses. Pulses 1 and 3 are respectively for the upper switches of the first and second arm. Pulses 2 and 4 are for the lower switches.
      | For a 3-arm  bridge: Six pulses. Pulses 1,3 and 5 are respectively for the upper switches of the first,second and third arm. Pulses 2,4 and 6 are for the lower switches.
      | For double 3-arm bridges: Twelve pulses.The first six pulses (pulses 1 to 6) must be sent to the first 3-arm bridge and the last six (pulses 7 to 12) to the second 3-arm bridge.
      | 
      | By selecting "Internal generation" you can can control the modulation index m, frequency and phase of the output voltage  from the internal parameters (m, Freq and Phase). Otherwise, external signals are used for pulse generation. The width of the input vector must be 1 for single phase bridges ( 1-arm or 2-arm)  and 3 for 3-phase bridges  (single or double bridge).
      mask TypeOptions GeneratorMode: 1-arm  bridge (2 pulses) | 2-arm  bridge (4 pulses) | 3-arm  bridge (6 pulses) | Double 3-arm  bridges (12 pulses)
      mask Callback Internal: %powericon('psbcallbacks',gcb,'Discrete PWM Generator',[]);
      mask Display: disp('')
  EPC Inverter Controller Outputs : Subsystem
  Ext(0) or Int(1) : Constant
  GD_Enable : Constant
  HIL Outputs : Subsystem
  Manual Switch : ManualSwitch  CurrentSetting=0
  Mux to Pulses1 : Subsystem
  Mux to Pulses2 : Subsystem
  Mux to Pulses3 : Subsystem
  Mux to Pulses4 : Subsystem
  Mux to Pulses5 : Subsystem
  Open Top : Subsystem
  PV Signal Mapping : Subsystem
  PWM to RTE PWM : Subsystem
  RTE Conversion1 : rteventslib/Signal Attributes/RTE Conversion  inputdatatype=Double  outputdatatype=RTE Boolean  compensation=Enabled  nbMaxEvents=4  sampleTime=Ts
  RTE Conversion2 : rteventslib/Signal Attributes/RTE Conversion  inputdatatype=RTE Boolean  outputdatatype=Double  compensation=Enabled  nbMaxEvents=4  sampleTime=Ts
  RTE Conversion3 : rteventslib/Signal Attributes/RTE Conversion  inputdatatype=RTE Boolean  outputdatatype=Double  compensation=Enabled  nbMaxEvents=4  sampleTime=Ts
  RTE Selector : Subsystem
  RTE Switch : rteventslib/Signal Routing/RTE Switch  switchType=u2 = Double; u1 u3 = RTE Boolean  criteria=u2 >= Threshold  threshold=0.5  interpolate=on  nbMaxEvents=4
  RTE_External2 : Constant  Value=0.1
  Signal Mapping : Subsystem
  Subtract : Sum  Inputs=+-
  Switch : Switch  Threshold=0.5
  BESS Precharge : Outport
  BESS DC Contactor : Outport  Port=2
  BESS MX1 Main AC : Outport  Port=3
  BESS MX2 Remote AC : Outport  Port=4
  BESS Gate Drive : Outport  Port=5
  BESS Gate Drive RTE : Outport  Port=6
  PWM : Outport  Port=7
  PV Precharge : Outport  Port=8
  PV DC Contactor : Outport  Port=9
  PV MX1 Main AC : Outport  Port=10
  PV MX2 Remote AC : Outport  Port=11
  PV Gate Drive : Outport  Port=12
  wires:
  RTE Conversion2/1 -> Mux to Pulses5/1(Mux_6_Pulses)
  Mux to Pulses5/7(Bus) -> PV Gate Drive/1
  Bus Selector1/2 -> PV DC Contactor/1  "<PV_K2_Main_DC>"
  Bus Selector1/1 -> PV Precharge/1  "<PV_K1_Precharge_DC>"
  EPC Inverter Controller Outputs/4(Digital Inputs) -> Bus Selector4/1, PWM to RTE PWM/1(PWM_in), Bus Selector1/1
  Bus Selector1/3 -> PV MX1 Main AC/1  "<PV_MX1_Main_AC>"
  Bus Selector1/4 -> PV MX2 Remote AC/1  "<PV_MX2_Remote_AC>"
  "PV HIL Output Inv Internal "/1 -> HIL Outputs/6(PV Inv Internal)
  PV HIL Outputs Local Sense/1 -> HIL Outputs/7(PV Local Sense)
  PV HIL Outputs Remote Sense/1 -> HIL Outputs/8(PV Remote Sense)
  PV Signal Mapping/1(TSD_RTE_v2) -> RTE Conversion2/1
  EPC Inverter Controller Outputs/7(PV_TSD_RTE) -> PV Signal Mapping/1(In1)
  BESS Signal Mapping/2(TSD_RTE_v2) -> [BESS_Ext_TSD]
  Demux1/3 -> Bus Creator4/3
  Demux1/5 -> Bus Creator4/5
  GD_Enable/1 -> Switch/2
  Demux1/1 -> Bus Creator4/1
  Demux1/2 -> Bus Creator4/2
  Bus Creator4/1 -> Switch/1
  All Open/1(Pulses8) -> Switch/3
  Demux1/4 -> Bus Creator4/4
  Demux1/6 -> Bus Creator4/6
  "BESS HIL Output Inv Internal "/1 -> HIL Outputs/1(BESS Inv Internal)
  Console Input/1 -> EPC Inverter Controller Outputs/1(Console Input)
  Constant Modulation/1 -> Discrete PWM Generator/1(Modulation)
  Ext(0) or Int(1)/1 -> Discrete PWM Generator/2(Ext(0) or Int(1))
  6-pulse RTE PWM generator (with deadtime)/1(RTE) -> [Int_RTE]
  RTE Conversion3/1 -> Mux to Pulses4/1(Mux_6_Pulses)
  Mux to Pulses4/7(Bus) -> Demux1/1
  Switch/1 -> BESS Gate Drive/1
  6-pulse RTE PWM generator (with deadtime)/2(SPS) -> Data Type Conversion/1
  Data Type Conversion/1 -> Subtract/1
  RTE_External2/1 -> Subtract/2
  Subtract/1 -> Mux to Pulses3/1(Mux_6_Pulses)
  Bus Selector4/2 -> BESS DC Contactor/1  "<BESS_K2_Main_DC>"
  Bus Selector4/1 -> BESS Precharge/1  "<BESS_K1_Precharge_DC>"
  EPC Inverter Controller Outputs/3(PWM) -> PWM/1
  RTE Conversion1/1 -> [Int_SinTri]
  Discrete PWM Generator/2(Pulses) -> RTE Conversion1/1, Mux to Pulses1/1(Mux_6_Pulses)
  [Int_SinTri] -> RTE Selector/3(In2)
  Open Top/1(Pulses6) -> RTE Selector/1(In0)
  [Int_RTE] -> RTE Selector/4(In3)
  En/1 -> Bus Selector/1, RTE Selector/6(En)
  [Ext_PWM] -> Manual Switch/1, RTE Selector/2(In1)
  RTE Selector/1(Out) -> Manual Switch/2
  Manual Switch/1 -> Mux to Pulses2/1(Mux_6_Pulses), RTE Conversion3/1, BESS Gate Drive RTE/1
  EPC Inverter Controller Outputs/5(PWM_RTE) -> Signal Mapping/1(In1)
  Signal Mapping/1(Out1) -> RTE Switch/3
  RTE Switch/1 -> [Ext_PWM]
  PWM to RTE PWM/1(RTE_PWM) -> RTE Switch/1
  Bus Selector/1 -> RTE Switch/2  "<Ext_PWM_RTE_Signal>"
  EPC Inverter Controller Outputs/6(BESS_TSD_RTE) -> BESS Signal Mapping/1(In1)
  [BESS_Ext_TSD] -> RTE Selector/5(In4)
  BESS HIL Outputs Local Sense/1 -> HIL Outputs/2(BESS Local Sense)
  BESS HIL Outputs Remote Sense/1 -> HIL Outputs/3(BESS Remote Sense)
  Bus Selector4/3 -> BESS MX1 Main AC/1  "<BESS_MX1_Main_AC>"
  Bus Selector4/4 -> BESS MX2 Remote AC/1  "<BESS_MX2_Remote_AC>"
  BESS HIL Outputs MX2 to MX1/1 -> HIL Outputs/4(BESS Inv MX2 to MX1 Sense)
  BESS HIL Outputs Inv filter/1 -> HIL Outputs/5(BESS Inv Filter)

== system BANSHEE/SS_PV_BESS/EPC/Inverter_Batt_RTE ==
  note: What does the maximum number of events mean for RTE?
      | What should this be set to?
  note: 1 e-4
      | 1.1 Vf
      | 10 Events
  note: Now 200 Events
  Gate_Drives_RTE : Inport
  Bus Creator1 : BusCreator  Inputs=7
  DC_Bus : powerlib/Elements/Parallel RLC Branch  LConnTagsString=a  RConnTagsString=__new0  BranchType=RC  Resistance=20e3  Inductance=1e-3  SetiL0=off  InitialCurrent=0  Capacitance=2*(925e-6)  Setx0=on  InitialVoltage=0  Measurements=None
  Inv1 : powerlib/Measurements/Current Measurement  PhasorSimulation=off  OutputType=Complex  PSBequivalent=0
  Inv2 : powerlib/Measurements/Current Measurement  PhasorSimulation=off  OutputType=Complex  PSBequivalent=0
  Inv3 : powerlib/Measurements/Current Measurement  PhasorSimulation=off  OutputType=Complex  PSBequivalent=0
  Inv_DC1 : powerlib/Measurements/Current Measurement  PhasorSimulation=off  OutputType=Complex  PSBequivalent=0
  Inv_DC2 : powerlib/Measurements/Current Measurement  PhasorSimulation=off  OutputType=Complex  PSBequivalent=0
  TSB_hiZ snubber_free (contains 6 real diode) : Subsystem
      mask Display: plot(0,0,100,100,[34,34],[60,90],[34,34],[20,50],[60,50],[60,60],[55,59,50,55],[60,50,50,60],[55,55,34],[50,34,34],[34,55,55],[75,75,60],[29,34],[57,50],[23,23,26,23,23,13],[55,51,55,58,55,55])
  V_DClink_1 : powerlib/Measurements/Voltage Measurement  PhasorSimulation=off  OutputType=Complex  PSBequivalent=0
  V_DClink_2 : powerlib/Measurements/Voltage Measurement  PhasorSimulation=off  OutputType=Complex  PSBequivalent=0
  Inv_1 : PMIOPort  Port=1  Side=Left
  Inv_2 : PMIOPort  Port=2  Side=Left
  Inv_3 : PMIOPort  Port=3  Side=Left
  DC+ : PMIOPort  Port=4  Side=Right
  DC- : PMIOPort  Port=5  Side=Right
  m : Outport
  wires:
  Gate_Drives_RTE/1 -> TSB_hiZ snubber_free (contains 6 real diode)/1(g)
  Inv3/1 -> [Inv_Ph3_W_Iout]
  Inv1/1 -> [Inv_Ph1_U_Iout]
  Inv2/1 -> [Inv_Ph2_V_Iout]
  V_DClink_1/1 -> [Inv_Vdc1]
  V_DClink_2/1 -> [Inv_Vdc2]
  Bus Creator1/1 -> m/1
  [Inv_Ph1_U_Iout] -> Bus Creator1/1  "Inv_1"
  [Inv_Ph2_V_Iout] -> Bus Creator1/2  "Inv_2"
  [Inv_Ph3_W_Iout] -> Bus Creator1/3  "Inv_3"
  [Inv_Idc1] -> Bus Creator1/4  "Inv_Idc1"
  [Inv_Idc2] -> Bus Creator1/5  "Inv_Idc2"
  [Inv_Vdc1] -> Bus Creator1/6  "Inv_Vdc1"
  [Inv_Vdc2] -> Bus Creator1/7  "Inv_Vdc2"
  Inv_DC1/1 -> [Inv_Idc1]
  Inv_DC2/1 -> [Inv_Idc2]
  connections:
  Inv_DC1/RConn1 -- TSB_hiZ snubber_free (contains 6 real diode)/RConn1
  TSB_hiZ snubber_free (contains 6 real diode)/LConn1 -- Inv1/RConn1
  TSB_hiZ snubber_free (contains 6 real diode)/LConn2 -- Inv2/RConn1
  TSB_hiZ snubber_free (contains 6 real diode)/LConn3 -- Inv3/RConn1
  DC_Bus/LConn1 -- Inv_DC2/RConn1 -- V_DClink_2/LConn1 -- Inv_DC1/LConn1 -- V_DClink_1/LConn1
  DC+/RConn1 -- Inv_DC2/LConn1
  Inv_1/RConn1 -- Inv1/LConn1
  Inv_2/RConn1 -- Inv2/LConn1
  Inv_3/RConn1 -- Inv3/LConn1
  DC-/RConn1 -- DC_Bus/RConn1 -- V_DClink_2/LConn2 -- TSB_hiZ snubber_free (contains 6 real diode)/RConn2 -- V_DClink_1/LConn2

== system BANSHEE/SS_PV_BESS/EPC/Inverter_Batt_RTE1 ==
  note: What does the maximum number of events mean for RTE?
      | What should this be set to?
  note: 1 e-4
      | 1.1 Vf
      | 10 Events
  note: Now 200 Events
  Gate_Drives_RTE : Inport
  Bus Creator1 : BusCreator  Inputs=7
  DC_Bus : powerlib/Elements/Parallel RLC Branch  LConnTagsString=a  RConnTagsString=__new0  BranchType=RC  Resistance=20e3  Inductance=1e-3  SetiL0=off  InitialCurrent=0  Capacitance=2*(925e-6)  Setx0=on  InitialVoltage=0  Measurements=None
  Inv1 : powerlib/Measurements/Current Measurement  PhasorSimulation=off  OutputType=Complex  PSBequivalent=0
  Inv2 : powerlib/Measurements/Current Measurement  PhasorSimulation=off  OutputType=Complex  PSBequivalent=0
  Inv3 : powerlib/Measurements/Current Measurement  PhasorSimulation=off  OutputType=Complex  PSBequivalent=0
  Inv_DC1 : powerlib/Measurements/Current Measurement  PhasorSimulation=off  OutputType=Complex  PSBequivalent=0
  Inv_DC2 : powerlib/Measurements/Current Measurement  PhasorSimulation=off  OutputType=Complex  PSBequivalent=0
  TSB_hiZ snubber_free (contains 6 real diode) : Subsystem
      mask Display: plot(0,0,100,100,[34,34],[60,90],[34,34],[20,50],[60,50],[60,60],[55,59,50,55],[60,50,50,60],[55,55,34],[50,34,34],[34,55,55],[75,75,60],[29,34],[57,50],[23,23,26,23,23,13],[55,51,55,58,55,55])
  V_DClink_1 : powerlib/Measurements/Voltage Measurement  PhasorSimulation=off  OutputType=Complex  PSBequivalent=0
  V_DClink_2 : powerlib/Measurements/Voltage Measurement  PhasorSimulation=off  OutputType=Complex  PSBequivalent=0
  Inv_1 : PMIOPort  Port=1  Side=Left
  Inv_2 : PMIOPort  Port=2  Side=Left
  Inv_3 : PMIOPort  Port=3  Side=Left
  DC+ : PMIOPort  Port=4  Side=Right
  DC- : PMIOPort  Port=5  Side=Right
  m : Outport
  wires:
  Gate_Drives_RTE/1 -> TSB_hiZ snubber_free (contains 6 real diode)/1(g)
  Inv3/1 -> [Inv_Ph3_W_Iout]
  Inv1/1 -> [Inv_Ph1_U_Iout]
  Inv2/1 -> [Inv_Ph2_V_Iout]
  V_DClink_1/1 -> [Inv_Vdc1]
  V_DClink_2/1 -> [Inv_Vdc2]
  Bus Creator1/1 -> m/1
  [Inv_Ph1_U_Iout] -> Bus Creator1/1  "Inv_1"
  [Inv_Ph2_V_Iout] -> Bus Creator1/2  "Inv_2"
  [Inv_Ph3_W_Iout] -> Bus Creator1/3  "Inv_3"
  [Inv_Idc1] -> Bus Creator1/4  "Inv_Idc1"
  [Inv_Idc2] -> Bus Creator1/5  "Inv_Idc2"
  [Inv_Vdc1] -> Bus Creator1/6  "Inv_Vdc1"
  [Inv_Vdc2] -> Bus Creator1/7  "Inv_Vdc2"
  Inv_DC1/1 -> [Inv_Idc1]
  Inv_DC2/1 -> [Inv_Idc2]
  connections:
  Inv_DC1/RConn1 -- TSB_hiZ snubber_free (contains 6 real diode)/RConn1
  TSB_hiZ snubber_free (contains 6 real diode)/LConn1 -- Inv1/RConn1
  TSB_hiZ snubber_free (contains 6 real diode)/LConn2 -- Inv2/RConn1
  TSB_hiZ snubber_free (contains 6 real diode)/LConn3 -- Inv3/RConn1
  DC_Bus/LConn1 -- Inv_DC2/RConn1 -- V_DClink_2/LConn1 -- Inv_DC1/LConn1 -- V_DClink_1/LConn1
  DC+/RConn1 -- Inv_DC2/LConn1
  Inv_1/RConn1 -- Inv1/LConn1
  Inv_2/RConn1 -- Inv2/LConn1
  Inv_3/RConn1 -- Inv3/LConn1
  DC-/RConn1 -- DC_Bus/RConn1 -- V_DClink_2/LConn2 -- TSB_hiZ snubber_free (contains 6 real diode)/RConn2 -- V_DClink_1/LConn2
